simulink model "HybridControllerD2D2onebay"  (R2019a)
settings: Solver=FixedStepDiscrete  StartTime=0.0  StopTime=inf  FixedStep=controlPeriod  RelTol=1e-3
PreLoadFcn:
  | initializeSimulation
  | initializeSCRAMNetGT
  | ATS_setup
values from neighbouring files (symbols this model uses):
  controlPeriod = 1/2048    (= 0.00048828125)    [initializeSimulation.m]
  nDOF = 2    [initializeSimulation.m]
undefined symbols (not defined in the file or in its folder): HybridCtrlParameters, MRC, nAct, Nl, node, P_range, Par, SN, Threshold, Zden, Znum
libraries: simulink x12, cwcec_scgt_lib x5, slrtlib x5, HybridSimLib x1
settings Model: ExtModeArmWhenConnect=off  Creator=mvetsch  LastModifiedBy=Andreas
settings DataIOCC: SaveFormat=Array  SaveOutput=off  SignalLogging=off  SaveTime=off  ReturnWorkspaceOutputs=off  SignalLoggingName=sigsOut
settings OptimizationCC: BlockReduction=off  OptimizeBlockIOStorage=off  BufferReuse=off  GlobalBufferReuse=off  ExpressionFolding=off  ExpressionDepthLimit=2147483647  LocalBlockOutputs=off  InitFltsAndDblsToZero=on  EfficientFloat2IntCast=on  LifeSpan=inf  SimCompilerOptimization=on  OptimizeDataStoreBuffers=off  BusAssignmentInplaceUpdate=off
settings DebuggingCC: SaveWithParameterizedLinksMsg=none  CheckSSInitialOutputMsg=off  UnderspecifiedInitializationDetection=Classic  MergeDetectMultiDrivingBlocksExec=none  AllowSymbolicDim=off  StateNameClashWarn=warning  PregeneratedLibrarySubsystemCodeDiagnostic=none  SFUnexpectedBacktrackingDiag=warning  SFNoUnconditionalDefaultTransitionDiag=warning  SFExecutionAtInitializationDiag=none  ArithmeticOperatorsInVariantConditions=warning
settings HardwareCC: ProdBitPerPointer=32  ProdBitPerSizeT=32  ProdBitPerPtrDiffT=32  ProdLargestAtomicFloat=None  ProdWordSize=32  ProdLongLongMode=on  ProdHWDeviceType=Generic->32-bit x86 compatible  TargetHWDeviceType=32-bit Generic
settings ModelReferenceCC: PropagateSignalLabelsOutOfModel=off
settings SFSimCC: SimCustomHeaderCode="#include \"PredictorCorrector.h\""  SimUserSources=PredictorCorrector.c  SimUserIncludeDirs="\"C:\\Program Files\\OpenFresco\\SourceCode\\SRC\\experimentalControl\\Simulink\\HybridSimToolbox\""  SimUseLocalCustomCode=off  SimParseCustomCode=off
settings RTWCC: SystemTargetFile=slrt.tlc  TemplateMakefile=slrt_default_tmf  Description=Simulink Real-Time  RTWUseLocalCustomCode=off  CustomHeaderCode="#include \"PredictorCorrector.h\""  CustomInclude="\"C:\\Program Files\\OpenFresco\\SourceCode\\SRC\\experimentalControl\\Simulink\\HybridSimToolbox\""  CustomSource=PredictorCorrector.c  CodeExecutionProfiling=on  RTWCompilerOptimization=on
settings CodeAppCC: StateflowObjectComments=on
settings SimulinkRealTimeCC: TargetFcnLib=ansi_tfl_tmw.mat  PreserveStateflowLocalDataDimensions=off  RL32IRQSourceModifier=Auto (PCI only)  xPCIRQSourceBoard=SCRAMNet_GT200
settings ConfigComp: CovMetricSettings=dw  CovHtmlReporting=on  CovSaveCumulativeToWorkspaceVar=on  CovSaveSingleToWorkspaceVar=on  CovExternalEMLEnable=off

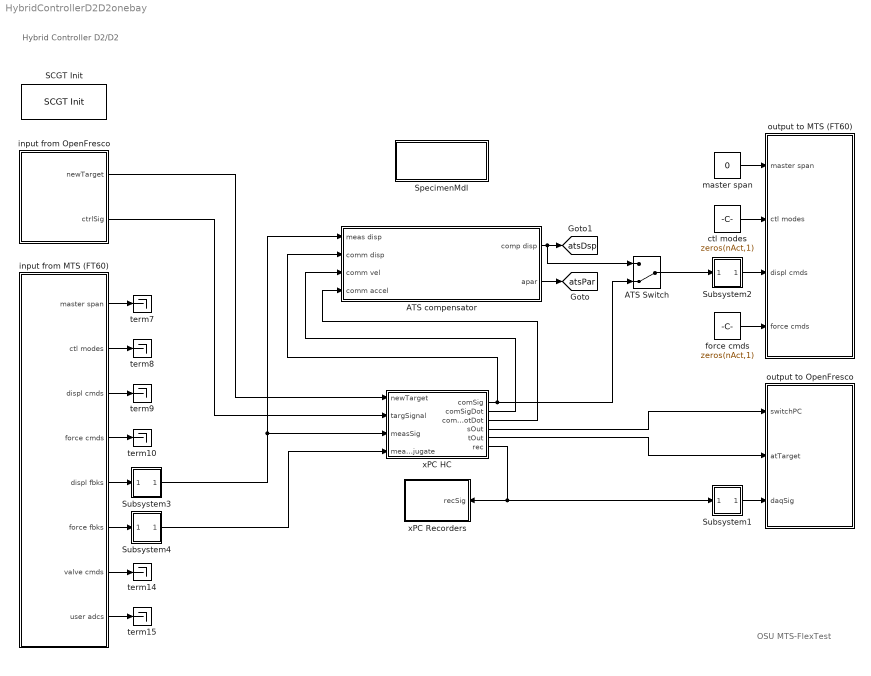
== system HybridControllerD2D2onebay ==
  note: Hybrid Controller D2/D2
  note: OSU MTS-FlexTest
  ATS Switch : ManualSwitch  CurrentSetting=0
  ATS compensator : Subsystem  mask{param=Par}
      mask prompts: param "Initial a0, a1, a2 values :"
  SCGT Init : cwcec_scgt_lib/SCGT Init   node=node  pci=-1
      settings: SourceProductName=Simulink Real-Time: SCRAMNetGT
  SpecimenMdl : Subsystem
      mask Display: fprintf('Test\nSpecimen');
  Subsystem1 : Subsystem
      mask Display: disp('I/O')
  Subsystem2 : Subsystem
      mask Display: disp('I/O')
  Subsystem3 : Subsystem
      mask Display: disp('I/O')
  Subsystem4 : Subsystem
      mask Display: disp('I/O')
  ctl modes : Constant  Value=zeros(nAct,1)
  force cmds : Constant  Value=zeros(nAct,1)
  input from MTS (FT60) : Subsystem
  input from OpenFresco : Subsystem
  master span : Constant  Value=0
  output to MTS (FT60) : Subsystem
  output to OpenFresco : Subsystem
  term{7..10,14..15} (6 alike) : Terminator
  xPC HC : Subsystem  mask(Hybrid Controller: D2/D2){nDOF=HybridCtrlParameters.nDOF, upFact=HybridCtrlParameters.upFact, dtInt=HybridCtrlParameters.dtInt, dtSim=HybridCtrlParameters.dtSim, dtCon=HybridCtrlParameters.dtCon, N=HybridCtrlParameters.N, iDelay=HybridCtrlParameters.iDelay}
      mask prompts: nDOF "Number of DOF: nDOF"; upFact "Upsample Factor: upFact"; dtInt "Integration time step: dtInt"; dtSim "Simulation time step: dtSim"; dtCon "Controller time step: dtCon"; N "Number of substeps: N"; iDelay "Number of delay steps: iDelay"
      mask help: Hybrid Controller using C0-continuous quadratic Lagrange interpolation for prediction and correction
      mask Display: disp('xPC Target\nHybrid Controller\n(D2/D2)')
  xPC Recorders : Subsystem  mask{nDOF=HybridCtrlParameters.nDOF}
      mask prompts: nDOF "Number of DOF: nDOF"
  tag scope: atsDsp=global, atsPar=global
  wires:
  input from MTS (FT60)/2(ctl modes) -> term8/1
  input from MTS (FT60)/4(force cmds) -> term10/1
  input from MTS (FT60)/7(valve cmds) -> term14/1
  input from MTS (FT60)/1(master span) -> term7/1
  master span/1 -> output to MTS (FT60)/1(master span)
  force cmds/1 -> output to MTS (FT60)/4(force cmds)
  ctl modes/1 -> output to MTS (FT60)/2(ctl modes)
  input from MTS (FT60)/3(displ cmds) -> term9/1
  input from OpenFresco/1(newTarget) -> xPC HC/1(newTarget)
  input from OpenFresco/2(ctrlSig) -> xPC HC/2(targSignal)
  xPC HC/1(comSig) -> ATS Switch/2, ATS compensator/2(comm disp)
  xPC HC/5(tOut) -> output to OpenFresco/2(atTarget)
  Subsystem1/1(Out1) -> output to OpenFresco/3(daqSig)
  input from MTS (FT60)/8(user adcs) -> term15/1
  xPC HC/4(sOut) -> output to OpenFresco/1(switchPC)
  xPC HC/6(rec) -> Subsystem1/1(In1), xPC Recorders/1(recSig)
  xPC HC/2(comSigDot) -> ATS compensator/3(comm vel)
  xPC HC/3(comSigDotDot) -> ATS compensator/4(comm accel)
  ATS compensator/2(apar) -> [atsPar]
  ATS compensator/1(comp disp) -> ATS Switch/1, [atsDsp]
  Subsystem3/1(Out1) -> xPC HC/3(measSig), ATS compensator/1(meas disp)
  input from MTS (FT60)/5(displ fbks) -> Subsystem3/1(In1)
  input from MTS (FT60)/6(force fbks) -> Subsystem4/1(In1)
  Subsystem4/1(Out1) -> xPC HC/4(measSigConjugate)
  Subsystem2/1(Out1) -> output to MTS (FT60)/3(displ cmds)
  ATS Switch/1 -> Subsystem2/1(In1)

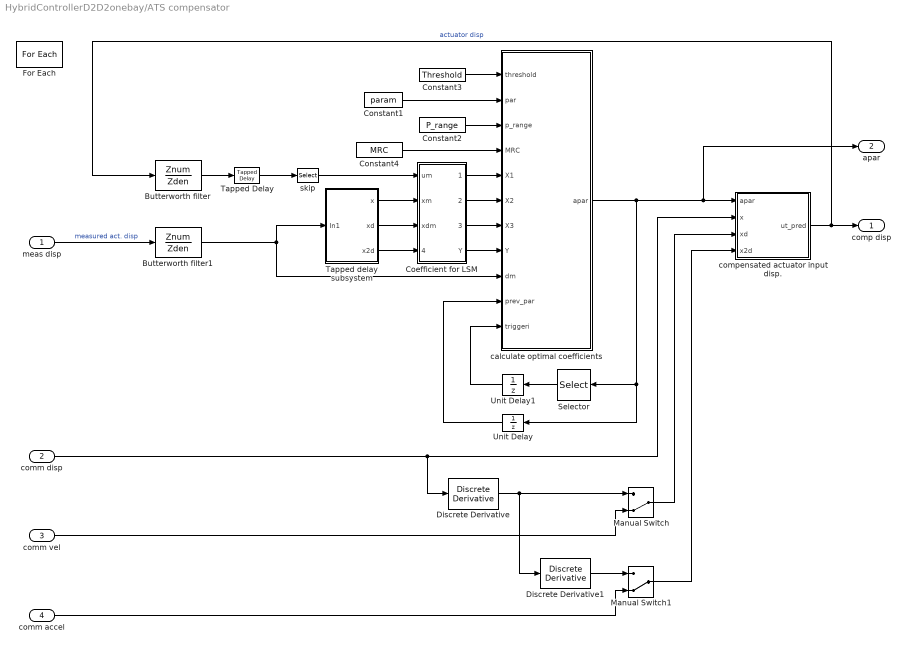
== system HybridControllerD2D2onebay/ATS compensator ==
  meas disp : Inport  Partition=on  PartitionDimension=1  PartitionWidth=1  PartitionOffset=0
  comm disp : Inport  Port=2  Partition=on  PartitionDimension=1  PartitionWidth=1  PartitionOffset=0
  comm vel : Inport  Port=3  Partition=on  PartitionDimension=1  PartitionWidth=1  PartitionOffset=0
  comm accel : Inport  Port=4  Partition=on  PartitionDimension=1  PartitionWidth=1  PartitionOffset=0
  Butterworth filter : DiscreteTransferFcn  Numerator=Znum  Denominator=Zden
  Butterworth filter1 : DiscreteTransferFcn  Numerator=Znum  Denominator=Zden
  Coefficient for LSM : Subsystem
  Constant1 : Constant  Value=param
  Constant2 : Constant  Value=P_range
  Constant3 : Constant  Value=Threshold
  Constant4 : Constant  Value=MRC
  Discrete Derivative : simulink/Discrete/Discrete Derivative  gainval=1.0  ICPrevScaledInput=0.0  OutMin=[]  OutMax=[]  OutDataType=fixdt(1, 16)  OutScaling=2^-10  DoSatur=off
  Discrete Derivative1 : simulink/Discrete/Discrete Derivative  gainval=1.0  ICPrevScaledInput=0.0  OutMin=[]  OutMax=[]  OutDataType=fixdt(1, 16)  OutScaling=2^-10  DoSatur=off
  For Each : ForEach  DisableCoverage=on  IterateSubsysMaskParameter=on  SubsysMaskParameterIterationDimension=2  IndexMode=One-based
  Manual Switch : ManualSwitch  CurrentSetting=0
  Manual Switch1 : ManualSwitch  CurrentSetting=0
  Selector : Selector  InputPortWidth=4  IndexOptions=Index vector (dialog)  Indices=4  OutputSizes=1
  Tapped Delay : simulink/Discrete/Tapped Delay  vinit=0.0  samptime=-1  NumDelays=Nl  DelayOrder=Oldest  includeCurrent=off
  Tapped delay subsystem : Subsystem
  Unit Delay : UnitDelay  SampleTime=-1  HasFrameUpgradeWarning=on
  Unit Delay1 : UnitDelay  SampleTime=-1  HasFrameUpgradeWarning=on
  calculate optimal coefficients : MATLAB Function  TreatAsAtomicUnit=on
  compensated actuator input disp. : MATLAB Function  TreatAsAtomicUnit=on
  skip : Selector  InputPortWidth=Nl  IndexOptions=Index vector (dialog)  Indices=[1:SN:Nl]  OutputSizes=1
  comp disp : Outport  ConcatenationDimension=1
  apar : Outport  Port=2  ConcatenationDimension=1
  wires:
  meas disp/1 -> Butterworth filter1/1  "measured act. disp"
  Tapped Delay/1 -> skip/1
  calculate optimal coefficients/1(apar) -> Unit Delay/1, Selector/1, apar/1, compensated actuator input disp./1(apar)
  compensated actuator input disp./1(ut_pred) -> comp disp/1, Butterworth filter/1  "actuator disp"
  Constant1/1 -> calculate optimal coefficients/2(par)
  Constant2/1 -> calculate optimal coefficients/3(p_range)
  Unit Delay/1 -> calculate optimal coefficients/10(prev_par)
  comm disp/1 -> compensated actuator input disp./2(x), Discrete Derivative/1
  skip/1 -> Coefficient for LSM/1(um)
  Tapped delay subsystem/1(x) -> Coefficient for LSM/2(xm)
  Tapped delay subsystem/2(xd) -> Coefficient for LSM/3(xdm)
  Tapped delay subsystem/3(x2d) -> Coefficient for LSM/4(x2dm)
  Coefficient for LSM/1(X(1,:)) -> calculate optimal coefficients/5(X1)
  Coefficient for LSM/2(X(2,:)) -> calculate optimal coefficients/6(X2)
  Coefficient for LSM/3(X(3,:)) -> calculate optimal coefficients/7(X3)
  Coefficient for LSM/4(Y) -> calculate optimal coefficients/8(Y)
  Unit Delay1/1 -> calculate optimal coefficients/11(triggeri)
  Constant3/1 -> calculate optimal coefficients/1(threshold)
  Butterworth filter/1 -> Tapped Delay/1
  Constant4/1 -> calculate optimal coefficients/4(MRC)
  Selector/1 -> Unit Delay1/1
  Manual Switch/1 -> compensated actuator input disp./3(xd)
  Discrete Derivative/1 -> Manual Switch/1, Discrete Derivative1/1
  comm vel/1 -> Manual Switch/2
  Discrete Derivative1/1 -> Manual Switch1/1
  Manual Switch1/1 -> compensated actuator input disp./4(x2d)
  comm accel/1 -> Manual Switch1/2
  Butterworth filter1/1 -> Tapped delay subsystem/1(In1), calculate optimal coefficients/9(dm)

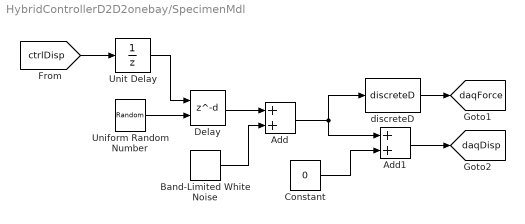
== system HybridControllerD2D2onebay/SpecimenMdl ==
  Add : Sum
  Add1 : Sum
  Band-Limited White Noise : simulink/Sources/Band-Limited White Noise  Cov=1e-7  Ts=controlPeriod  seed=[23341]
  Constant : Constant  Value=0
  Delay : Delay  DelayLengthSource=Input port  DelayLengthUpperLimit=20
      settings: InputPortMap=u0,p1
  Uniform Random Number : UniformRandomNumber  Minimum=0  Maximum=2  SampleTime=controlPeriod
  Unit Delay : UnitDelay  SampleTime=-1  HasFrameUpgradeWarning=on
  discreteD : HybridSimLib/Material Models/discreteD  k=2.8  fy=1.5  alpha=0.01  beta=0.5  gamma=0.5  n=2  dt=controlPeriod
      settings: SourceProductName=Hybrid Simulation
  tag scope: daqDisp=global, daqForce=global
  wires:
  discreteD/1 -> [daqForce]
  Add/1 -> Add1/1, discreteD/1
  Delay/1 -> Add/1
  Band-Limited White Noise/1 -> Add/2
  Uniform Random Number/1 -> Delay/2
  [ctrlDisp] -> Unit Delay/1
  Unit Delay/1 -> Delay/1
  Add1/1 -> [daqDisp]
  Constant/1 -> Add1/2

== system HybridControllerD2D2onebay/Subsystem1 ==
  In1 : Inport
  extract3 : Subsystem  mask(from Actuators){id=[4*nDOF+1:6*nDOF], size=5+8*nDOF}
      mask prompts: id "Index Vector: id"; size "Vector Size: size"
      mask help: To select from which actuator(s) the signals are coming from
      mask Display: disp('Extract')
  Out1 : Outport
  wires:
  In1/1 -> extract3/1(In1)
  extract3/1(Out1) -> Out1/1

== system HybridControllerD2D2onebay/Subsystem2 ==
  In1 : Inport
  Saturation : Saturate  UpperLimit=5  LowerLimit=-5
  assemble3 : Subsystem  mask(to Actuators){id=[1], size=nAct}
      mask prompts: id "Index Vector: id"; size "Vector Size: size"
      mask help: To select to which actuator(s) the signals are going to
      mask Display: disp('Assemble')
  Out1 : Outport
  tag scope: ctrlDisp=global
  wires:
  In1/1 -> [ctrlDisp], assemble3/1(In1)
  assemble3/1(Out1) -> Saturation/1
  Saturation/1 -> Out1/1

== system HybridControllerD2D2onebay/Subsystem3 ==
  In1 : Inport
  MovingAverage Filter : DiscreteFir  Coefficients=1/numSample*ones(1,numSample)  mask(Moving Average Filter){numSample=1}
      mask prompts: numSample "Number of Samples: numSample"
      mask help:
      | Moving average filter by using discrete FIR filter.
      | Set numSample = 1 for no filtering.
      mask Display: fprintf('MovingAvg\nFilter')
  extract5 : Subsystem  mask(from Actuators){id=[1], size=nAct}
      mask prompts: id "Index Vector: id"; size "Vector Size: size"
      mask help: To select from which actuator(s) the signals are coming from
      mask Display: disp('Extract')
  Out1 : Outport
  wires:
  extract5/1(Out1) -> MovingAverage Filter/1
  In1/1 -> extract5/1(In1)
  [daqDisp] -> Out1/1

== system HybridControllerD2D2onebay/Subsystem4 ==
  In1 : Inport
  MovingAverage Filter1 : DiscreteFir  Coefficients=1/numSample*ones(1,numSample)  mask(Moving Average Filter){numSample=1}
      mask prompts: numSample "Number of Samples: numSample"
      mask help:
      | Moving average filter by using discrete FIR filter.
      | Set numSample = 1 for no filtering.
      mask Display: fprintf('MovingAvg\nFilter')
  extract6 : Subsystem  mask(from Actuators){id=[1], size=nAct}
      mask prompts: id "Index Vector: id"; size "Vector Size: size"
      mask help: To select from which actuator(s) the signals are coming from
      mask Display: disp('Extract')
  Out1 : Outport
  wires:
  In1/1 -> extract6/1(In1)
  extract6/1(Out1) -> MovingAverage Filter1/1
  [daqForce] -> Out1/1

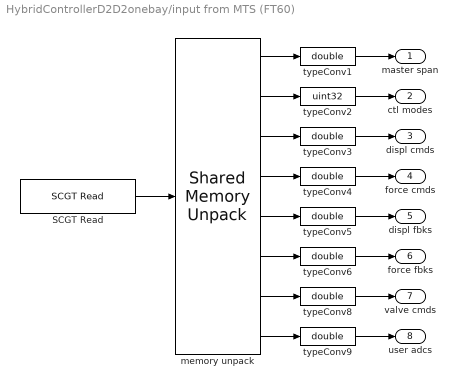
== system HybridControllerD2D2onebay/input from MTS (FT60) ==
  SCGT Read : cwcec_scgt_lib/SCGT Read   partition=node.Partitions(5:12)  ts=controlPeriod  pci=-1
      settings: SourceProductName=Simulink Real-Time: SCRAMNetGT
  memory unpack : slrtlib/Shared Memory/Shared Memory Unpack   partition=node.Partitions(5:12)
      settings: SourceProductName=Simulink Real-Time  SourceProductBaseCode=XP
  typeConv{1,3..6,8..9} (7 alike) : DataTypeConversion  OutDataTypeStr=double  SaturateOnIntegerOverflow=on  RndMeth=Zero
  typeConv2 : DataTypeConversion  OutDataTypeStr=uint32  SaturateOnIntegerOverflow=on  RndMeth=Zero
  master span : Outport
  ctl modes : Outport  Port=2
  displ cmds : Outport  Port=3
  force cmds : Outport  Port=4
  displ fbks : Outport  Port=5
  force fbks : Outport  Port=6
  valve cmds : Outport  Port=7
  user adcs : Outport  Port=8
  wires:
  typeConv9/1 -> user adcs/1
  typeConv8/1 -> valve cmds/1
  typeConv6/1 -> force fbks/1
  typeConv5/1 -> displ fbks/1
  typeConv4/1 -> force cmds/1
  typeConv3/1 -> displ cmds/1
  typeConv1/1 -> master span/1
  SCGT Read/1 -> memory unpack/1
  typeConv2/1 -> ctl modes/1
  memory unpack/1 -> typeConv1/1
  memory unpack/2 -> typeConv2/1
  memory unpack/3 -> typeConv3/1
  memory unpack/4 -> typeConv4/1
  memory unpack/5 -> typeConv5/1
  memory unpack/6 -> typeConv6/1
  memory unpack/8 -> typeConv9/1
  memory unpack/7 -> typeConv8/1

== system HybridControllerD2D2onebay/input from OpenFresco ==
  "SCGT Read " : cwcec_scgt_lib/SCGT Read   partition=node.Partitions(13:14)  ts=controlPeriod  pci=-1
      settings: SourceProductName=Simulink Real-Time: SCRAMNetGT
  memory unpack : slrtlib/Shared Memory/Shared Memory Unpack   partition=node.Partitions(13:14)
      settings: SourceProductName=Simulink Real-Time  SourceProductBaseCode=XP
  typeConv2 : DataTypeConversion  OutDataTypeStr=double  SaturateOnIntegerOverflow=on  RndMeth=Zero
  newTarget : Outport
  ctrlSig : Outport  Port=2
  wires:
  typeConv2/1 -> ctrlSig/1
  "SCGT Read "/1 -> memory unpack/1
  memory unpack/2 -> typeConv2/1
  memory unpack/1 -> newTarget/1

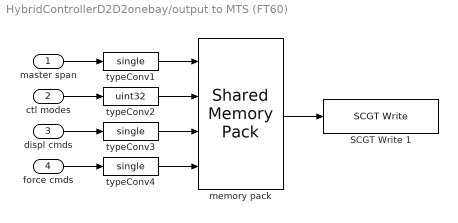
== system HybridControllerD2D2onebay/output to MTS (FT60) ==
  master span : Inport
  ctl modes : Inport  Port=2
  displ cmds : Inport  Port=3
  force cmds : Inport  Port=4
  SCGT Write 1 : cwcec_scgt_lib/SCGT Write   partition=node.Partitions(1:4)  ts=controlPeriod  pci=-1
      settings: SourceProductName=Simulink Real-Time: SCRAMNetGT
  memory pack : slrtlib/Shared Memory/Shared Memory Pack   partition=node.Partitions(1:4)
      settings: SourceProductName=Simulink Real-Time  SourceProductBaseCode=XP
  typeConv1 : DataTypeConversion  OutDataTypeStr=single  SaturateOnIntegerOverflow=on  RndMeth=Zero
  typeConv2 : DataTypeConversion  OutDataTypeStr=uint32  SaturateOnIntegerOverflow=on  RndMeth=Zero
  typeConv3 : DataTypeConversion  OutDataTypeStr=single  SaturateOnIntegerOverflow=on  RndMeth=Zero
  typeConv4 : DataTypeConversion  OutDataTypeStr=single  SaturateOnIntegerOverflow=on  RndMeth=Zero
  wires:
  force cmds/1 -> typeConv4/1
  master span/1 -> typeConv1/1
  memory pack/1 -> SCGT Write 1/1
  displ cmds/1 -> typeConv3/1
  ctl modes/1 -> typeConv2/1
  typeConv1/1 -> memory pack/1
  typeConv2/1 -> memory pack/2
  typeConv3/1 -> memory pack/3
  typeConv4/1 -> memory pack/4

== system HybridControllerD2D2onebay/output to OpenFresco ==
  switchPC : Inport
  atTarget : Inport  Port=2
  daqSig : Inport  Port=3
  SC150 pack : slrtlib/Shared Memory/Shared Memory Pack   partition=node.Partitions(15:17)
      settings: SourceProductName=Simulink Real-Time  SourceProductBaseCode=XP
  "SCGT Write " : cwcec_scgt_lib/SCGT Write   partition=node.Partitions(15:17)  ts=controlPeriod  pci=-1
      settings: SourceProductName=Simulink Real-Time: SCRAMNetGT
  typeConv3 : DataTypeConversion  OutDataTypeStr=single  SaturateOnIntegerOverflow=on  RndMeth=Zero
  wires:
  daqSig/1 -> typeConv3/1
  SC150 pack/1 -> "SCGT Write "/1
  atTarget/1 -> SC150 pack/2
  switchPC/1 -> SC150 pack/1
  typeConv3/1 -> SC150 pack/3

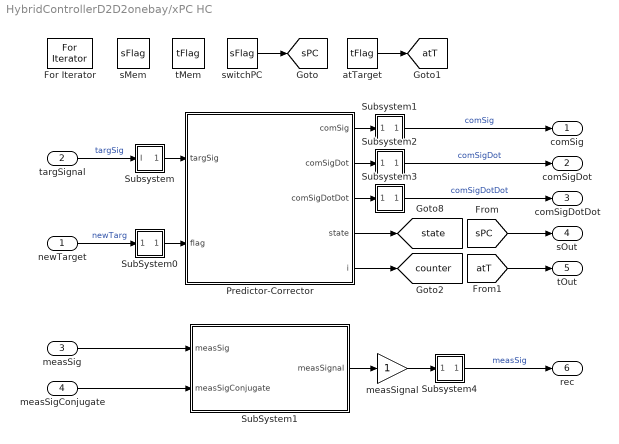
== system HybridControllerD2D2onebay/xPC HC ==
  newTarget : Inport
  targSignal : Inport  Port=2
  measSig : Inport  Port=3
  measSigConjugate : Inport  Port=4
  For Iterator : ForIterator  IterationLimit=upFact  ShowIterationPort=off
  Predictor-Corrector : Stateflow chart  TreatAsAtomicUnit=on
  SubSystem0 : Subsystem
      mask Display: disp('I/O')
  SubSystem1 : Subsystem
  Subsystem : Subsystem
      mask Display: disp('I/O')
  Subsystem1 : Subsystem
      mask Display: disp('I/O')
  Subsystem2 : Subsystem
      mask Display: disp('I/O')
  Subsystem3 : Subsystem
      mask Display: disp('I/O')
  Subsystem4 : Subsystem
      mask Display: disp('I/O')
  atTarget : DataStoreRead  DataStoreName=tFlag
  measSignal : Gain  OutDataTypeStr=double
  sMem : DataStoreMemory  DataStoreName=sFlag  ShowAdditionalParam=off  OutDataTypeStr=int32
  switchPC : DataStoreRead  DataStoreName=sFlag
  tMem : DataStoreMemory  DataStoreName=tFlag  ShowAdditionalParam=off  OutDataTypeStr=int32
  comSig : Outport
  comSigDot : Outport  Port=2
  comSigDotDot : Outport  Port=3
  sOut : Outport  Port=4
  tOut : Outport  Port=5
  rec : Outport  Port=6
  tag scope: atT=global, counter=global, sPC=global, state=global
  wires:
  measSignal/1 -> Subsystem4/1(measSig)
  SubSystem1/1(measSignal) -> measSignal/1
  Predictor-Corrector/5(i) -> [counter]
  SubSystem0/1(Out) -> Predictor-Corrector/2(flag)
  newTarget/1 -> SubSystem0/1(In)  "newTarg"
  switchPC/1 -> [sPC]
  atTarget/1 -> [atT]
  Subsystem/1(O) -> Predictor-Corrector/1(targSig)
  measSig/1 -> SubSystem1/1(measSig)
  measSigConjugate/1 -> SubSystem1/2(measSigConjugate)
  Predictor-Corrector/1(comSig) -> Subsystem1/1(In)
  Predictor-Corrector/2(comSigDot) -> Subsystem2/1(In)
  Predictor-Corrector/3(comSigDotDot) -> Subsystem3/1(In)
  targSignal/1 -> Subsystem/1(I)  "targSig"
  Predictor-Corrector/4(state) -> [state]
  Subsystem2/1(Out) -> comSigDot/1  "comSigDot"
  Subsystem3/1(Out) -> comSigDotDot/1  "comSigDotDot"
  Subsystem1/1(Out) -> comSig/1  "comSig"
  Subsystem4/1(Out1) -> rec/1  "measSig"
  [sPC] -> sOut/1
  [atT] -> tOut/1

== system HybridControllerD2D2onebay/xPC Recorders ==
  recSig : Inport
  Demux : Demux  Outputs=[(4*nDOF) (4*nDOF) 5]
  Mux : Mux  Inputs=5
  Scope (xPC) 1 : slrtlib/Displays and Logging/Scope   scopeno=1  scopetype=File  autostart=on  viewmode=Numerical  formatstr='%15.6f'  grid=on  ylimits=[-4,4]  nosamples=60*1024  noprepostsamples=0  interleave=1  triggermode=FreeRun  triggersignal=1  trigsignalfromport=off  triggerlevel=0.0  triggerslope=Either  triggerscope=1  triggersample=0  filename=H:\xpcRec.dat  mode=Lazy  writesize=512  autorestart=on  dynamicfilemode=off  maxwritefilesize=512*1024^2
  wires:
  recSig/1 -> Demux/1
  [atsDsp] -> Mux/2
  [atsPar] -> Mux/4
  Demux/1 -> Mux/1
  Demux/2 -> Mux/3
  Mux/1 -> Scope (xPC) 1/1
  Demux/3 -> Mux/5

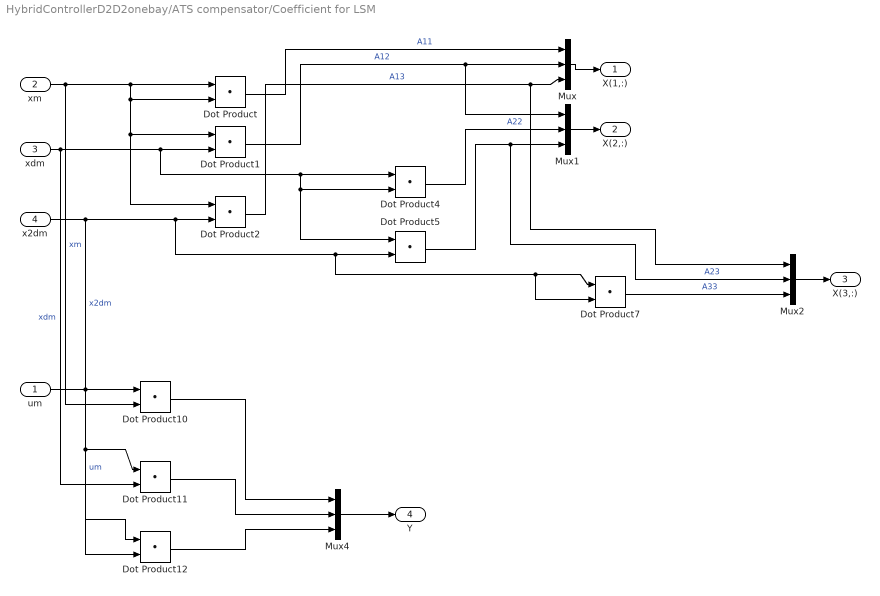
== system HybridControllerD2D2onebay/ATS compensator/Coefficient for LSM ==
  um : Inport
  xm : Inport  Port=2
  xdm : Inport  Port=3
  x2dm : Inport  Port=4
  Dot Product{,1..2,4..5,7,10..12} (9 alike) : DotProduct  InputSameDT=on  OutDataTypeStr=Inherit: Inherit via internal rule
  Mux{,1..2,4} (4 alike) : Mux  Inputs=3
  X(1,:) : Outport
  X(2,:) : Outport  Port=2
  X(3,:) : Outport  Port=3
  Y : Outport  Port=4
  wires:
  xm/1 -> Dot Product/1, Dot Product/2, Dot Product1/1, Dot Product2/1, Dot Product10/2  "xm"
  xdm/1 -> Dot Product1/2, Dot Product4/1, Dot Product4/2, Dot Product5/1, Dot Product11/2  "xdm"
  x2dm/1 -> Dot Product2/2, Dot Product5/2, Dot Product7/1, Dot Product7/2, Dot Product12/2  "x2dm"
  um/1 -> Dot Product10/1, Dot Product11/1, Dot Product12/1  "um"
  Dot Product/1 -> Mux/1  "A11"
  Dot Product1/1 -> Mux/2, Mux1/1  "A12"
  Dot Product2/1 -> Mux/3, Mux2/1  "A13"
  Mux/1 -> X(1,:)/1
  Dot Product4/1 -> Mux1/2  "A22"
  Dot Product5/1 -> Mux1/3, Mux2/2  "A23"
  Mux1/1 -> X(2,:)/1
  Dot Product7/1 -> Mux2/3  "A33"
  Mux2/1 -> X(3,:)/1
  Mux4/1 -> Y/1
  Dot Product10/1 -> Mux4/1
  Dot Product11/1 -> Mux4/2
  Dot Product12/1 -> Mux4/3

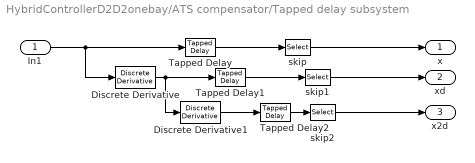
== system HybridControllerD2D2onebay/ATS compensator/Tapped delay subsystem ==
  In1 : Inport
  Discrete Derivative : simulink/Discrete/Discrete Derivative  gainval=1.0  ICPrevScaledInput=0.0  OutMin=[]  OutMax=[]  OutDataType=fixdt(1, 16)  OutScaling=2^-10  DoSatur=off
  Discrete Derivative1 : simulink/Discrete/Discrete Derivative  gainval=1.0  ICPrevScaledInput=0.0  OutMin=[]  OutMax=[]  OutDataType=fixdt(1, 16)  OutScaling=2^-10  DoSatur=off
  Tapped Delay : simulink/Discrete/Tapped Delay  vinit=0.0  samptime=-1  NumDelays=Nl  DelayOrder=Oldest  includeCurrent=off
  Tapped Delay1 : simulink/Discrete/Tapped Delay  vinit=0.0  samptime=-1  NumDelays=Nl  DelayOrder=Oldest  includeCurrent=off
  Tapped Delay2 : simulink/Discrete/Tapped Delay  vinit=0.0  samptime=-1  NumDelays=Nl  DelayOrder=Oldest  includeCurrent=off
  skip : Selector  InputPortWidth=Nl  IndexOptions=Index vector (dialog)  Indices=[1:SN:Nl]  OutputSizes=1
  skip1 : Selector  InputPortWidth=Nl  IndexOptions=Index vector (dialog)  Indices=[1:SN:Nl]  OutputSizes=1
  skip2 : Selector  InputPortWidth=Nl  IndexOptions=Index vector (dialog)  Indices=[1:SN:Nl]  OutputSizes=1
  x : Outport
  xd : Outport  Port=2
  x2d : Outport  Port=3
  wires:
  In1/1 -> Discrete Derivative/1, Tapped Delay/1
  Discrete Derivative/1 -> Discrete Derivative1/1, Tapped Delay1/1
  Discrete Derivative1/1 -> Tapped Delay2/1
  Tapped Delay/1 -> skip/1
  Tapped Delay1/1 -> skip1/1
  Tapped Delay2/1 -> skip2/1
  skip/1 -> x/1
  skip1/1 -> xd/1
  skip2/1 -> x2d/1

== system HybridControllerD2D2onebay/Subsystem1/extract3 ==
  In1 : Inport
  Selector : Selector  InputPortWidth=size  IndexOptions=Index vector (dialog)  Indices=id  OutputSizes=1
  Out1 : Outport
  wires:
  Selector/1 -> Out1/1
  In1/1 -> Selector/1

== system HybridControllerD2D2onebay/Subsystem2/assemble3 ==
  In1 : Inport
  Assignment : Assignment  OutputInitialize=Specify size for each dimension in table  IndexOptions=Index vector (port)  Indices=1  OutputSizes=size
  Constant : Constant  Value=id
  Out1 : Outport
  wires:
  Constant/1 -> Assignment/2
  Assignment/1 -> Out1/1
  In1/1 -> Assignment/1

== system HybridControllerD2D2onebay/Subsystem3/extract5 ==
  In1 : Inport
  Selector : Selector  InputPortWidth=size  IndexOptions=Index vector (dialog)  Indices=id  OutputSizes=1
  Out1 : Outport
  wires:
  Selector/1 -> Out1/1
  In1/1 -> Selector/1

== system HybridControllerD2D2onebay/Subsystem4/extract6 ==
  In1 : Inport
  Selector : Selector  InputPortWidth=size  IndexOptions=Index vector (dialog)  Indices=id  OutputSizes=1
  Out1 : Outport
  wires:
  Selector/1 -> Out1/1
  In1/1 -> Selector/1

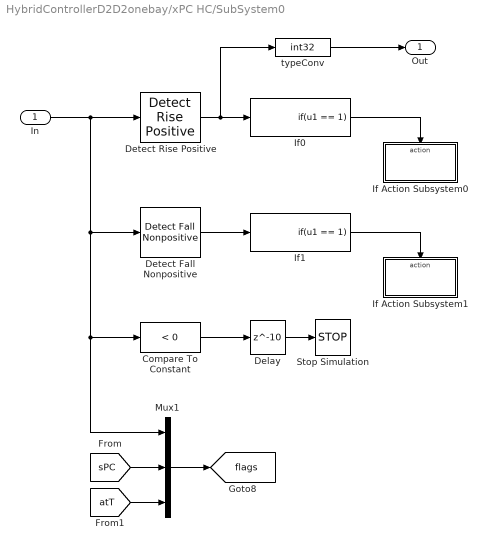
== system HybridControllerD2D2onebay/xPC HC/SubSystem0 ==
  In : Inport
  Compare To Constant : simulink/Logic and Bit Operations/Compare To Constant  relop=<  const=0  OutDataTypeStr=boolean
  Delay : Delay  DelayLength=10
  Detect Fall Nonpositive : simulink/Logic and Bit Operations/Detect Fall Nonpositive  vinit=0  OutDataTypeStr=uint8
      settings: SourceProductName=Simulink  SourceProductBaseCode=SL
  Detect Rise Positive : simulink/Logic and Bit Operations/Detect Rise Positive  vinit=0  OutDataTypeStr=uint8
  If Action Subsystem0 : Subsystem  TreatAsAtomicUnit=on
  If Action Subsystem1 : Subsystem  TreatAsAtomicUnit=on
  If0 : If  IfExpression=u1 == 1  ShowElse=off
  If1 : If  IfExpression=u1 == 1  ShowElse=off
  Mux1 : Mux  Inputs=3
  Stop Simulation : Stop
  typeConv : DataTypeConversion  OutDataTypeStr=int32  SaturateOnIntegerOverflow=on  RndMeth=Zero
  Out : Outport
  tag scope: flags=global
  wires:
  Detect Rise Positive/1 -> If0/1, typeConv/1
  Detect Fall Nonpositive/1 -> If1/1
  If1/1 -> If Action Subsystem1/Action
  If0/1 -> If Action Subsystem0/Action
  typeConv/1 -> Out/1
  Mux1/1 -> [flags]
  [sPC] -> Mux1/2
  [atT] -> Mux1/3
  In/1 -> Detect Rise Positive/1, Detect Fall Nonpositive/1, Compare To Constant/1, Mux1/1
  Compare To Constant/1 -> Delay/1
  Delay/1 -> Stop Simulation/1

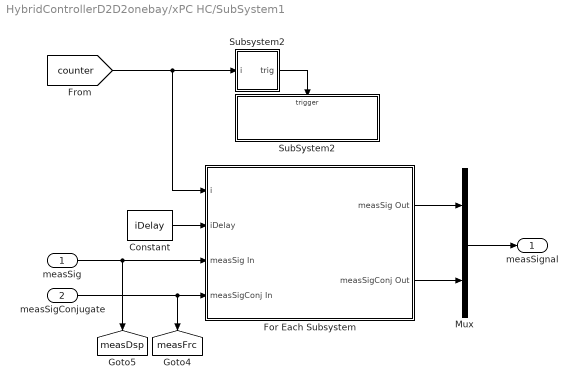
== system HybridControllerD2D2onebay/xPC HC/SubSystem1 ==
  measSig : Inport
  measSigConjugate : Inport  Port=2
  Constant : Constant  Value=iDelay
  For Each Subsystem : Subsystem  TreatAsAtomicUnit=on
  Mux : Mux  Inputs=2
  SubSystem2 : Subsystem  TreatAsAtomicUnit=on
  Subsystem2 : Subsystem
  measSignal : Outport
  tag scope: measDsp=global, measFrc=global
  wires:
  Subsystem2/1(trig) -> SubSystem2/Trigger
  [counter] -> Subsystem2/1(i), For Each Subsystem/1(i)
  Constant/1 -> For Each Subsystem/2(iDelay)
  measSig/1 -> For Each Subsystem/3(measSig In), [measDsp]
  measSigConjugate/1 -> For Each Subsystem/4(measSigConj In), [measFrc]
  For Each Subsystem/1(measSig Out) -> Mux/1
  For Each Subsystem/2(measSigConj Out) -> Mux/2
  Mux/1 -> measSignal/1

== system HybridControllerD2D2onebay/xPC HC/Subsystem ==
  I : Inport  PortDimensions=nDOF
  Dummy Aug : Mux  Inputs=[nDOF 1]
  Dummy Zero : Constant  Value=0  OutDataTypeStr=double  SampleTime=-1
  O : Outport  PortDimensions=nDOF+1
  tag scope: targSig=global
  wires:
  Dummy Zero/1 -> Dummy Aug/2
  I/1 -> Dummy Aug/1, [targSig]
  Dummy Aug/1 -> O/1

== system HybridControllerD2D2onebay/xPC HC/Subsystem1 ==
  In : Inport  PortDimensions=nDOF+1
  Dummy Trn : Demux  Outputs=[nDOF 1]
  Terminator3 : Terminator
  Out : Outport  PortDimensions=nDOF
  tag scope: comSig=global
  wires:
  Dummy Trn/2 -> Terminator3/1
  Dummy Trn/1 -> Out/1, [comSig]
  In/1 -> Dummy Trn/1

== system HybridControllerD2D2onebay/xPC HC/Subsystem2 ==
  In : Inport  PortDimensions=nDOF+1
  Dummy Trn : Demux  Outputs=[nDOF 1]
  Terminator3 : Terminator
  Out : Outport  PortDimensions=nDOF
  tag scope: comSigDot=global
  wires:
  Dummy Trn/2 -> Terminator3/1
  Dummy Trn/1 -> Out/1, [comSigDot]
  In/1 -> Dummy Trn/1

== system HybridControllerD2D2onebay/xPC HC/Subsystem3 ==
  In : Inport  PortDimensions=nDOF+1
  Dummy Trn : Demux  Outputs=[nDOF 1]
  Terminator3 : Terminator
  Out : Outport  PortDimensions=nDOF
  tag scope: comSigDotDot=global
  wires:
  Dummy Trn/2 -> Terminator3/1
  Dummy Trn/1 -> Out/1, [comSigDotDot]
  In/1 -> Dummy Trn/1

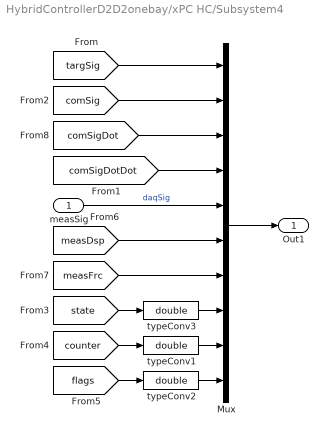
== system HybridControllerD2D2onebay/xPC HC/Subsystem4 ==
  measSig : Inport
  Mux : Mux  Inputs=10
  typeConv1 : DataTypeConversion  OutDataTypeStr=double  SaturateOnIntegerOverflow=on  RndMeth=Zero
  typeConv2 : DataTypeConversion  OutDataTypeStr=double  SaturateOnIntegerOverflow=on  RndMeth=Zero
  typeConv3 : DataTypeConversion  OutDataTypeStr=double  SaturateOnIntegerOverflow=on  RndMeth=Zero
  Out1 : Outport
  wires:
  measSig/1 -> Mux/5  "daqSig"
  [flags] -> typeConv2/1
  [counter] -> typeConv1/1
  [state] -> typeConv3/1
  typeConv3/1 -> Mux/8
  typeConv1/1 -> Mux/9
  typeConv2/1 -> Mux/10
  [measFrc] -> Mux/7
  [measDsp] -> Mux/6
  [comSigDotDot] -> Mux/4
  [comSigDot] -> Mux/3
  [comSig] -> Mux/2
  [targSig] -> Mux/1
  Mux/1 -> Out1/1

== system HybridControllerD2D2onebay/xPC HC/SubSystem0/If Action Subsystem0 ==
  Action Port : ActionPort  PropagateVarSize=During execution  ActionPortLabel=if(u1 == 1)
  Data Store Write0 : DataStoreWrite  DataStoreName=sFlag
  Data Store Write1 : DataStoreWrite  DataStoreName=tFlag
  atTargetFlag : Constant  Value=0  OutDataTypeStr=int32  SampleTime=-1
  switchFlag : Constant  OutDataTypeStr=int32  SampleTime=-1
  wires:
  atTargetFlag/1 -> Data Store Write1/1
  switchFlag/1 -> Data Store Write0/1

== system HybridControllerD2D2onebay/xPC HC/SubSystem0/If Action Subsystem1 ==
  Action Port : ActionPort  PropagateVarSize=During execution  ActionPortLabel=if(u1 == 1)
  Data Store Write0 : DataStoreWrite  DataStoreName=sFlag
  switchFlag : Constant  Value=0  OutDataTypeStr=int32  SampleTime=-1
  wires:
  switchFlag/1 -> Data Store Write0/1

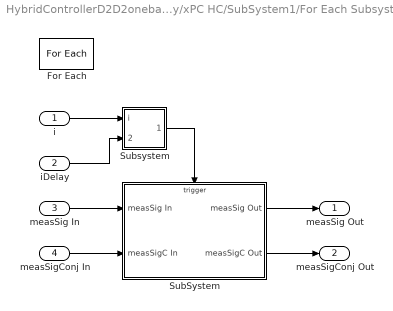
== system HybridControllerD2D2onebay/xPC HC/SubSystem1/For Each Subsystem ==
  i : Inport
  iDelay : Inport  Port=2  Partition=on  PartitionDimension=1  PartitionWidth=1  PartitionOffset=0
  measSig In : Inport  Port=3  Partition=on  PartitionDimension=1  PartitionWidth=1  PartitionOffset=0
  measSigConj In : Inport  Port=4  Partition=on  PartitionDimension=1  PartitionWidth=1  PartitionOffset=0
  For Each : ForEach  DisableCoverage=on  IndexMode=One-based
  SubSystem : Subsystem  TreatAsAtomicUnit=on
  Subsystem : Subsystem
  measSig Out : Outport  ConcatenationDimension=1
  measSigConj Out : Outport  Port=2  ConcatenationDimension=1
  wires:
  Subsystem/1(trig) -> SubSystem/Trigger
  measSig In/1 -> SubSystem/1(measSig In)
  measSigConj In/1 -> SubSystem/2(measSigC In)
  SubSystem/1(measSig Out) -> measSig Out/1
  SubSystem/2(measSigC Out) -> measSigConj Out/1
  iDelay/1 -> Subsystem/2(iDelay)
  i/1 -> Subsystem/1(i)

== system HybridControllerD2D2onebay/xPC HC/SubSystem1/SubSystem2 ==
  Trigger : TriggerPort  VariantControl=(inherit)
  Data Store Write : DataStoreWrite  DataStoreName=tFlag
  atTargetFlag : Constant  OutDataTypeStr=int32  SampleTime=-1
  wires:
  atTargetFlag/1 -> Data Store Write/1

== system HybridControllerD2D2onebay/xPC HC/SubSystem1/Subsystem2 ==
  i : Inport
  Add : Sum
  Constant : Constant  Value=max(iDelay)
  Constant1 : Constant  Value=N
  If : If  IfExpression=u1 == 0
  If Action Subsystem1 : Subsystem  TreatAsAtomicUnit=on
  If Action Subsystem2 : Subsystem  TreatAsAtomicUnit=on
  trig : Outport
  wires:
  Constant/1 -> If/1, If Action Subsystem2/2(In2)
  If/1 -> If Action Subsystem1/Action
  If/2 -> If Action Subsystem2/Action
  If Action Subsystem1/1(Out1) -> Add/1
  If Action Subsystem2/1(Out1) -> Add/2
  Add/1 -> trig/1
  i/1 -> If Action Subsystem1/2(In2), If Action Subsystem2/1(In1)
  Constant1/1 -> If Action Subsystem1/1(In1)

== system HybridControllerD2D2onebay/xPC HC/SubSystem1/For Each Subsystem/SubSystem ==
  measSig In : Inport
  measSigC In : Inport  Port=2
  Trigger : TriggerPort  VariantControl=(inherit)
  measSig Out : Outport  InitialOutput=[0]
  measSigC Out : Outport  Port=2  InitialOutput=[0]
  wires:
  measSigC In/1 -> measSigC Out/1
  measSig In/1 -> measSig Out/1

== system HybridControllerD2D2onebay/xPC HC/SubSystem1/For Each Subsystem/Subsystem ==
  i : Inport
  iDelay : Inport  Port=2
  Add : Sum
  Constant1 : Constant  Value=N
  If : If  IfExpression=u1 == 0
  If Action Subsystem1 : Subsystem  TreatAsAtomicUnit=on
  If Action Subsystem2 : Subsystem  TreatAsAtomicUnit=on
  trig : Outport
  wires:
  iDelay/1 -> If/1, If Action Subsystem2/2(In2)
  If/1 -> If Action Subsystem1/Action
  If/2 -> If Action Subsystem2/Action
  If Action Subsystem1/1(Out1) -> Add/1
  If Action Subsystem2/1(Out1) -> Add/2
  Add/1 -> trig/1
  i/1 -> If Action Subsystem1/2(In2), If Action Subsystem2/1(In1)
  Constant1/1 -> If Action Subsystem1/1(In1)

== system HybridControllerD2D2onebay/xPC HC/SubSystem1/Subsystem2/If Action Subsystem1 ==
  In1 : Inport
  In2 : Inport  Port=2
  Action Port : ActionPort  ActionPortLabel=if(u1 == 0)
  Relational Operator : RelationalOperator  Operator===  OutDataTypeStr=boolean  RndMeth=Nearest
  Out1 : Outport  InitialOutput=0
  wires:
  Relational Operator/1 -> Out1/1
  In1/1 -> Relational Operator/1
  In2/1 -> Relational Operator/2

== system HybridControllerD2D2onebay/xPC HC/SubSystem1/Subsystem2/If Action Subsystem2 ==
  In1 : Inport
  In2 : Inport  Port=2
  Action Port : ActionPort  ActionPortLabel=else
  Relational Operator : RelationalOperator  Operator===  OutDataTypeStr=boolean  RndMeth=Nearest
  Out1 : Outport  InitialOutput=0
  wires:
  Relational Operator/1 -> Out1/1
  In1/1 -> Relational Operator/1
  In2/1 -> Relational Operator/2

== system HybridControllerD2D2onebay/xPC HC/SubSystem1/For Each Subsystem/Subsystem/If Action Subsystem1 ==
  In1 : Inport
  In2 : Inport  Port=2
  Action Port : ActionPort  ActionPortLabel=if(u1 == 0)
  Relational Operator : RelationalOperator  Operator===  OutDataTypeStr=boolean  RndMeth=Nearest
  Out1 : Outport  InitialOutput=0
  wires:
  Relational Operator/1 -> Out1/1
  In1/1 -> Relational Operator/1
  In2/1 -> Relational Operator/2

== system HybridControllerD2D2onebay/xPC HC/SubSystem1/For Each Subsystem/Subsystem/If Action Subsystem2 ==
  In1 : Inport
  In2 : Inport  Port=2
  Action Port : ActionPort  ActionPortLabel=else
  Relational Operator : RelationalOperator  Operator===  OutDataTypeStr=boolean  RndMeth=Nearest
  Out1 : Outport  InitialOutput=0
  wires:
  Relational Operator/1 -> Out1/1
  In1/1 -> Relational Operator/1
  In2/1 -> Relational Operator/2

== stateflow chart HybridControllerD2D2onebay/xPC HC/Predictor-Corrector ==
  state HybridController [parallel]
    settings: executionOrder=1
    state Initialize
      en:
      state = -1;
      i = 0; iSD = 0; diSD = 1;
      initData(nDOF,dtCon,dtSim,dtInt);
      state GetSetpoint
        en:
        setData(targSig);
        setSig(comSig,targSig);
        zeroSig(comSigDot);
        zeroSig(comSigDotDot);
        du:
        i = 0;
      (default) -> GetSetpoint
      GetSetpoint -> GetSetpoint : [after(dtCon,sec)]
          | {i=N}
    state Correct
      en:
      state = 0;
      setCurSig(comSig,i/N);
      setNewSig(targSig);
      en, du:
      di = min(max(diSD+1/(0.1*N)*(i-iSD),0.001),1.0);
      i = min(i+di,N);
      correctD2(comSig,i/N);
      correctV2(comSigDot,i/N);
      correctA2(comSigDotDot,i/N);
    state Predict
      en:
      state = 1;
      setCurSig(comSig,1.0);
      i = 1; iSD = 0; diSD = 1;
      du:
      i++;
      en, du:
      predictD2(comSig,i/N);
      predictV2(comSigDot,i/N);
      predictA2(comSigDotDot,i/N);
    state AutoSlowDown
      en:
      state = 2;
      en, du:
      diSD = 9-i/(0.1*N); i += diSD; iSD = i;
      predictD2(comSig,i/N);
      predictV2(comSigDot,i/N);
      predictA2(comSigDotDot,i/N);
    Correct -> Predict [order 1] : [flag==0 && i==N]
    (default) -> Initialize
    Initialize -> Correct : [flag==1]
        | {i=0}
    Predict -> Correct [order 2] : [flag==1]
    Predict -> AutoSlowDown [order 1] : [flag==0 && i>=0.8*N]
    AutoSlowDown -> Correct : [flag==1]
    Correct -> Correct [order 2] : [flag==1]
        | {i=0; iSD=0; diSD=1}
  data: targSig input double size=nDOF+1; flag input int32; comSig output double size=nDOF+1; comSigDot output double size=nDOF+1; comSigDotDot output double size=nDOF+1; state output int32; i output double; N parameter int32; nDOF parameter int32; di local double; diSD local double; iSD local double; dtCon parameter double; dtSim parameter double; dtInt parameter double

== matlab function HybridControllerD2D2onebay/ATS compensator/calculate optimal coefficients ==
  data: threshold input; par input; p_range input; MRC input; X1 input; apar output; X2 input; X3 input; Y input; dm input; prev_par input; triggeri input
function apar = fcn(threshold,par,p_range,MRC,X1,X2,X3,Y,dm,prev_par,triggeri)
%#codegen
%triggero=triggeri;
apar = [par; triggeri];

if( abs( dm ) > threshold || apar(4) )
    apar(4)=1;
    
    X = [X1 X2 X3];       
    
    temp=X\Y; 
    
    apar(1:3)=temp;
    
    if( isnan( apar(1) ) + isnan( apar(2) ) + isnan( apar(3) ) )
        apar=[par; triggeri];
    end
    
    
    % maximum change of rate
    if( abs(apar(1)-prev_par(1)) > MRC(1) )
        apar(1) = prev_par(1) + sign(apar(1)-prev_par(1))*MRC(1);
    end
    if( abs(apar(2)-prev_par(2)) > MRC(2) )
        apar(2) = prev_par(2) + sign(apar(2)-prev_par(2))*MRC(2);
    end
    if( abs(apar(3)-prev_par(3)) > MRC(3) )
        apar(3) = prev_par(3) + sign(apar(3)-prev_par(3))*MRC(3);
    end
    
    % limit of coefficients
    if( apar(1) < p_range(1,1) )
        apar(1) = p_range(1,1);
    end
    
    if( apar(1) > p_range(1,2) )
        apar(1) = p_range(1,2);
    end
    
    if( apar(2) < p_range(2,1) )
        apar(2) = p_range(2,1);
    end
    
    if( apar(2) > p_range(2,2) )
        apar(2) = p_range(2,2);
    end
    
    if( apar(3) < p_range(3,1) )
        apar(3) = p_range(3,1);
    end
    
    if( apar(3) > p_range(3,2) )
        apar(3) = p_range(3,2);
    end    
    
end

== matlab function HybridControllerD2D2onebay/ATS compensator/compensated actuator input disp. ==
  data: apar input; x input; xd input; x2d input; ut_pred output
function ut_pred = fcn(apar,x,xd,x2d)
%#codegen

ut_pred = apar(1)*x + apar(2)*xd + apar(3)*x2d;
